simulink model "bike_model_v1_20190513_oldmodel"  (R2016b)
settings: Solver=ode23s  StartTime=0.0  StopTime=sim_time  FixedStep=Ts_IMU  MaxStep=Ts  RelTol=1e-3
values from neighbouring files (symbols this model uses):
  A = [0      0            1 ... (first row only)    [bike_init_v1_20190523_oldmodel_NOfeedback_RealModelComparison.m]    (also in bike_init_v1_20190524_oldmodel_positionfeedback_Nobalancing.m; bike_init_v1_20190527_oldmodel_NObalancing.m; bike_init_v1_20190527_oldmodel_positionfeedback_and_indicator.m; bike_init_v1_20190528_oldmodel_positionfeedback_and_indicator.m)
  B = [0; 1; (a_real*v*sin(lambda_real))/(h_real*b_real)]    [bike_init_v1_20190523_oldmodel_NOfeedback_RealModelComparison.m]    (also in bike_init_v1_20190524_oldmodel_positionfeedback_Nobalancing.m; bike_init_v1_20190527_oldmodel_NObalancing.m; bike_init_v1_20190527_oldmodel_positionfeedback_and_indicator.m; bike_init_v1_20190528_oldmodel_positionfeedback_and_indicator.m)
  b_model = 1.095*(1+(-0.1+(0.2*rand)))    [bike_init_v1_20190523_oldmodel_NOfeedback_RealModelComparison.m]    (also in bike_init_v1_20190524_oldmodel_positionfeedback_Nobalancing.m = 1.095; bike_init_v1_20190527_oldmodel_NObalancing.m = 1.095; bike_init_v1_20190527_oldmodel_positionfeedback_and_indicator.m = 1.095; bike_init_v1_20190528_oldmodel_positionfeedback_and_indicator.m = 1.095)
  b_real = 1.095    [bike_init_v1_20190523_oldmodel_NOfeedback_RealModelComparison.m]    (also in bike_init_v1_20190524_oldmodel_positionfeedback_Nobalancing.m; bike_init_v1_20190527_oldmodel_NObalancing.m; bike_init_v1_20190527_oldmodel_positionfeedback_and_indicator.m; bike_init_v1_20190528_oldmodel_positionfeedback_and_indicator.m)
  complementary = 0.985    [bike_init_v1_20190523_oldmodel_NOfeedback_RealModelComparison.m]    (also in bike_init_v1_20190524_oldmodel_positionfeedback_Nobalancing.m; bike_init_v1_20190527_oldmodel_NObalancing.m; bike_init_v1_20190527_oldmodel_positionfeedback_and_indicator.m; bike_init_v1_20190528_oldmodel_positionfeedback_and_indicator.m)
  cumulative_dist_along_path = [0;cumsum(dist_from_vertex_to_vertex,1)]    [bike_init_v1_20190523_oldmodel_NOfeedback_RealModelComparison.m]    (also in bike_init_v1_20190524_oldmodel_positionfeedback_Nobalancing.m; bike_init_v1_20190527_oldmodel_NObalancing.m; bike_init_v1_20190527_oldmodel_positionfeedback_and_indicator.m; bike_init_v1_20190528_oldmodel_positionfeedback_and_indicator.m)
  damp = 0.4    [bike_init_v1_20190523_oldmodel_NOfeedback_RealModelComparison.m]    (also in bike_init_v1_20190524_oldmodel_positionfeedback_Nobalancing.m; bike_init_v1_20190527_oldmodel_NObalancing.m; bike_init_v1_20190527_oldmodel_positionfeedback_and_indicator.m; bike_init_v1_20190528_oldmodel_positionfeedback_and_indicator.m)
  Dead_Band = [0.055,-0.055,0.005]    [bike_init_v1_20190523_oldmodel_NOfeedback_RealModelComparison.m]    (also in bike_init_v1_20190524_oldmodel_positionfeedback_Nobalancing.m; bike_init_v1_20190527_oldmodel_NObalancing.m; bike_init_v1_20190527_oldmodel_positionfeedback_and_indicator.m; bike_init_v1_20190528_oldmodel_positionfeedback_and_indicator.m)
  delay = 0.045    [bike_init_v1_20190523_oldmodel_NOfeedback_RealModelComparison.m]    (also in bike_init_v1_20190524_oldmodel_positionfeedback_Nobalancing.m; bike_init_v1_20190527_oldmodel_NObalancing.m; bike_init_v1_20190527_oldmodel_positionfeedback_and_indicator.m; bike_init_v1_20190528_oldmodel_positionfeedback_and_indicator.m)
  delta_control = 1    [bike_init_v1_20190523_oldmodel_NOfeedback_RealModelComparison.m]    (also in bike_init_v1_20190524_oldmodel_positionfeedback_Nobalancing.m; bike_init_v1_20190527_oldmodel_NObalancing.m; bike_init_v1_20190527_oldmodel_positionfeedback_and_indicator.m; bike_init_v1_20190528_oldmodel_positionfeedback_and_indicator.m)
  direct_control = 1    [bike_init_v1_20190523_oldmodel_NOfeedback_RealModelComparison.m]    (also in bike_init_v1_20190524_oldmodel_positionfeedback_Nobalancing.m; bike_init_v1_20190527_oldmodel_NObalancing.m; bike_init_v1_20190527_oldmodel_positionfeedback_and_indicator.m; bike_init_v1_20190528_oldmodel_positionfeedback_and_indicator.m)
  filter_model = 1    [bike_init_v1_20190523_oldmodel_NOfeedback_RealModelComparison.m]    (also in bike_init_v1_20190524_oldmodel_positionfeedback_Nobalancing.m; bike_init_v1_20190527_oldmodel_NObalancing.m; bike_init_v1_20190527_oldmodel_positionfeedback_and_indicator.m; bike_init_v1_20190528_oldmodel_positionfeedback_and_indicator.m)
  forward_motor_dynamics = 0    [bike_init_v1_20190523_oldmodel_NOfeedback_RealModelComparison.m]    (also in bike_init_v1_20190524_oldmodel_positionfeedback_Nobalancing.m; bike_init_v1_20190527_oldmodel_NObalancing.m; bike_init_v1_20190527_oldmodel_positionfeedback_and_indicator.m; bike_init_v1_20190528_oldmodel_positionfeedback_and_indicator.m)
  fr_oscil = 1    [bike_init_v1_20190523_oldmodel_NOfeedback_RealModelComparison.m]    (also in bike_init_v1_20190524_oldmodel_positionfeedback_Nobalancing.m; bike_init_v1_20190527_oldmodel_NObalancing.m; bike_init_v1_20190527_oldmodel_positionfeedback_and_indicator.m; bike_init_v1_20190528_oldmodel_positionfeedback_and_indicator.m)
  g = 9.81    [bike_init_v1_20190523_oldmodel_NOfeedback_RealModelComparison.m]    (also in bike_init_v1_20190524_oldmodel_positionfeedback_Nobalancing.m; bike_init_v1_20190527_oldmodel_NObalancing.m; bike_init_v1_20190527_oldmodel_positionfeedback_and_indicator.m; bike_init_v1_20190528_oldmodel_positionfeedback_and_indicator.m)
  gain = 0.3    [bike_init_v1_20190523_oldmodel_NOfeedback_RealModelComparison.m]    (also in bike_init_v1_20190524_oldmodel_positionfeedback_Nobalancing.m; bike_init_v1_20190527_oldmodel_NObalancing.m; bike_init_v1_20190527_oldmodel_positionfeedback_and_indicator.m; bike_init_v1_20190528_oldmodel_positionfeedback_and_indicator.m)
  IMU_height_model = 0.45*(1+(-0.1+(0.2*rand)))    [bike_init_v1_20190523_oldmodel_NOfeedback_RealModelComparison.m]    (also in bike_init_v1_20190524_oldmodel_positionfeedback_Nobalancing.m = 0.45; bike_init_v1_20190527_oldmodel_NObalancing.m = 0.45; bike_init_v1_20190527_oldmodel_positionfeedback_and_indicator.m = 0.45; bike_init_v1_20190528_oldmodel_positionfeedback_and_indicator.m = 0.45)
  IMU_height_real = 0.45    [bike_init_v1_20190523_oldmodel_NOfeedback_RealModelComparison.m]    (also in bike_init_v1_20190524_oldmodel_positionfeedback_Nobalancing.m; bike_init_v1_20190527_oldmodel_NObalancing.m; bike_init_v1_20190527_oldmodel_positionfeedback_and_indicator.m; bike_init_v1_20190528_oldmodel_positionfeedback_and_indicator.m)
  initial_states = [deg2rad(0) deg2rad(0) deg2rad(0)]    [bike_init_v1_20190523_oldmodel_NOfeedback_RealModelComparison.m]    (also in bike_init_v1_20190524_oldmodel_positionfeedback_Nobalancing.m; bike_init_v1_20190527_oldmodel_NObalancing.m; bike_init_v1_20190527_oldmodel_positionfeedback_and_indicator.m; bike_init_v1_20190528_oldmodel_positionfeedback_and_indicator.m = [deg2rad(1) deg2rad(0) deg2rad(0)])
  initial_x = path_x(1)+x_ini_diff    [bike_init_v1_20190523_oldmodel_NOfeedback_RealModelComparison.m]    (also in bike_init_v1_20190524_oldmodel_positionfeedback_Nobalancing.m; bike_init_v1_20190527_oldmodel_NObalancing.m; bike_init_v1_20190527_oldmodel_positionfeedback_and_indicator.m; bike_init_v1_20190528_oldmodel_positionfeedback_and_indicator.m)
  initial_y = radius+y_ini_diff    (= 20)    [bike_init_v1_20190523_oldmodel_NOfeedback_RealModelComparison.m]    (also in bike_init_v1_20190524_oldmodel_positionfeedback_Nobalancing.m; bike_init_v1_20190527_oldmodel_NObalancing.m; bike_init_v1_20190527_oldmodel_positionfeedback_and_indicator.m; bike_init_v1_20190528_oldmodel_positionfeedback_and_indicator.m)
  input_velocity = 2    [bike_init_v1_20190523_oldmodel_NOfeedback_RealModelComparison.m]    (also in bike_init_v1_20190524_oldmodel_positionfeedback_Nobalancing.m = 2.5; bike_init_v1_20190527_oldmodel_NObalancing.m = 2.5; bike_init_v1_20190527_oldmodel_positionfeedback_and_indicator.m = 3; bike_init_v1_20190528_oldmodel_positionfeedback_and_indicator.m = 7)
  K_full_dis = zeros(length(velocity_lqr),3)    [bike_init_v1_20190523_oldmodel_NOfeedback_RealModelComparison.m]    (also in bike_init_v1_20190524_oldmodel_positionfeedback_Nobalancing.m; bike_init_v1_20190527_oldmodel_NObalancing.m; bike_init_v1_20190527_oldmodel_positionfeedback_and_indicator.m; bike_init_v1_20190528_oldmodel_positionfeedback_and_indicator.m)
  lambda_model = deg2rad(70)*(1+(-0.1+(0.2*rand)))    [bike_init_v1_20190523_oldmodel_NOfeedback_RealModelComparison.m]    (also in bike_init_v1_20190524_oldmodel_positionfeedback_Nobalancing.m = deg2rad(70); bike_init_v1_20190527_oldmodel_NObalancing.m = deg2rad(70); bike_init_v1_20190527_oldmodel_positionfeedback_and_indicator.m = deg2rad(70); bike_init_v1_20190528_oldmodel_positionfeedback_and_indicator.m = deg2rad(70))
  lambda_real = deg2rad(70)    [bike_init_v1_20190523_oldmodel_NOfeedback_RealModelComparison.m]    (also in bike_init_v1_20190524_oldmodel_positionfeedback_Nobalancing.m; bike_init_v1_20190527_oldmodel_NObalancing.m; bike_init_v1_20190527_oldmodel_positionfeedback_and_indicator.m; bike_init_v1_20190528_oldmodel_positionfeedback_and_indicator.m)
  lat_control = 1    [bike_init_v1_20190523_oldmodel_NOfeedback_RealModelComparison.m]    (also in bike_init_v1_20190524_oldmodel_positionfeedback_Nobalancing.m; bike_init_v1_20190527_oldmodel_NObalancing.m; bike_init_v1_20190527_oldmodel_positionfeedback_and_indicator.m; bike_init_v1_20190528_oldmodel_positionfeedback_and_indicator.m)
  look_ahead = 0    [bike_init_v1_20190523_oldmodel_NOfeedback_RealModelComparison.m]    (also in bike_init_v1_20190524_oldmodel_positionfeedback_Nobalancing.m; bike_init_v1_20190527_oldmodel_NObalancing.m; bike_init_v1_20190527_oldmodel_positionfeedback_and_indicator.m; bike_init_v1_20190528_oldmodel_positionfeedback_and_indicator.m)
  max_handlebar = 40*(pi/180)    (= 0.698131700798)    [bike_init_v1_20190523_oldmodel_NOfeedback_RealModelComparison.m]    (also in bike_init_v1_20190524_oldmodel_positionfeedback_Nobalancing.m; bike_init_v1_20190527_oldmodel_NObalancing.m; bike_init_v1_20190527_oldmodel_positionfeedback_and_indicator.m; bike_init_v1_20190528_oldmodel_positionfeedback_and_indicator.m)
  max_roll = pi/2    (= 1.57079632679)    [bike_init_v1_20190523_oldmodel_NOfeedback_RealModelComparison.m]    (also in bike_init_v1_20190524_oldmodel_positionfeedback_Nobalancing.m; bike_init_v1_20190527_oldmodel_NObalancing.m; bike_init_v1_20190527_oldmodel_positionfeedback_and_indicator.m; bike_init_v1_20190528_oldmodel_positionfeedback_and_indicator.m)
  max_steering_motor_acc = inf    [bike_init_v1_20190523_oldmodel_NOfeedback_RealModelComparison.m]    (also in bike_init_v1_20190524_oldmodel_positionfeedback_Nobalancing.m; bike_init_v1_20190527_oldmodel_NObalancing.m; bike_init_v1_20190527_oldmodel_positionfeedback_and_indicator.m; bike_init_v1_20190528_oldmodel_positionfeedback_and_indicator.m)
  max_steering_motor_speed = 7.5    [bike_init_v1_20190523_oldmodel_NOfeedback_RealModelComparison.m]    (also in bike_init_v1_20190524_oldmodel_positionfeedback_Nobalancing.m; bike_init_v1_20190527_oldmodel_NObalancing.m; bike_init_v1_20190527_oldmodel_positionfeedback_and_indicator.m; bike_init_v1_20190528_oldmodel_positionfeedback_and_indicator.m)
  min_handlebar = -max_handlebar    (= -0.698131700798)    [bike_init_v1_20190523_oldmodel_NOfeedback_RealModelComparison.m]    (also in bike_init_v1_20190524_oldmodel_positionfeedback_Nobalancing.m; bike_init_v1_20190527_oldmodel_NObalancing.m; bike_init_v1_20190527_oldmodel_positionfeedback_and_indicator.m; bike_init_v1_20190528_oldmodel_positionfeedback_and_indicator.m)
  min_roll = - max_roll    (= -1.57079632679)    [bike_init_v1_20190523_oldmodel_NOfeedback_RealModelComparison.m]    (also in bike_init_v1_20190524_oldmodel_positionfeedback_Nobalancing.m; bike_init_v1_20190527_oldmodel_NObalancing.m; bike_init_v1_20190527_oldmodel_positionfeedback_and_indicator.m; bike_init_v1_20190528_oldmodel_positionfeedback_and_indicator.m)
  min_steering_motor_acc = -inf    [bike_init_v1_20190523_oldmodel_NOfeedback_RealModelComparison.m]    (also in bike_init_v1_20190524_oldmodel_positionfeedback_Nobalancing.m; bike_init_v1_20190527_oldmodel_NObalancing.m; bike_init_v1_20190527_oldmodel_positionfeedback_and_indicator.m; bike_init_v1_20190528_oldmodel_positionfeedback_and_indicator.m)
  min_steering_motor_speed = -7.5    [bike_init_v1_20190523_oldmodel_NOfeedback_RealModelComparison.m]    (also in bike_init_v1_20190524_oldmodel_positionfeedback_Nobalancing.m; bike_init_v1_20190527_oldmodel_NObalancing.m; bike_init_v1_20190527_oldmodel_positionfeedback_and_indicator.m; bike_init_v1_20190528_oldmodel_positionfeedback_and_indicator.m)
  noise = 1    [bike_init_v1_20190523_oldmodel_NOfeedback_RealModelComparison.m]    (also in bike_init_v1_20190524_oldmodel_positionfeedback_Nobalancing.m; bike_init_v1_20190527_oldmodel_NObalancing.m; bike_init_v1_20190527_oldmodel_positionfeedback_and_indicator.m; bike_init_v1_20190528_oldmodel_positionfeedback_and_indicator.m)
  noise_encoder = 1e-7    (= 1e-07)    [bike_init_v1_20190523_oldmodel_NOfeedback_RealModelComparison.m]    (also in bike_init_v1_20190524_oldmodel_positionfeedback_Nobalancing.m; bike_init_v1_20190527_oldmodel_NObalancing.m; bike_init_v1_20190527_oldmodel_positionfeedback_and_indicator.m; bike_init_v1_20190528_oldmodel_positionfeedback_and_indicator.m)
  noise_hall = 0    [bike_init_v1_20190523_oldmodel_NOfeedback_RealModelComparison.m]    (also in bike_init_v1_20190524_oldmodel_positionfeedback_Nobalancing.m = 0.01; bike_init_v1_20190527_oldmodel_NObalancing.m; bike_init_v1_20190527_oldmodel_positionfeedback_and_indicator.m = 0.01; bike_init_v1_20190528_oldmodel_positionfeedback_and_indicator.m = 0.01)
  oscillations_roll = 0    [bike_init_v1_20190523_oldmodel_NOfeedback_RealModelComparison.m]    (also in bike_init_v1_20190524_oldmodel_positionfeedback_Nobalancing.m; bike_init_v1_20190527_oldmodel_NObalancing.m; bike_init_v1_20190527_oldmodel_positionfeedback_and_indicator.m; bike_init_v1_20190528_oldmodel_positionfeedback_and_indicator.m)
  oscillations_steer = 0    [bike_init_v1_20190523_oldmodel_NOfeedback_RealModelComparison.m]    (also in bike_init_v1_20190524_oldmodel_positionfeedback_Nobalancing.m; bike_init_v1_20190527_oldmodel_NObalancing.m; bike_init_v1_20190527_oldmodel_positionfeedback_and_indicator.m; bike_init_v1_20190528_oldmodel_positionfeedback_and_indicator.m)
  parameters_model = [g h_model b_model a_model lambda_model c_model]    [bike_init_v1_20190523_oldmodel_NOfeedback_RealModelComparison.m]    (also in bike_init_v1_20190524_oldmodel_positionfeedback_Nobalancing.m; bike_init_v1_20190527_oldmodel_NObalancing.m; bike_init_v1_20190527_oldmodel_positionfeedback_and_indicator.m; bike_init_v1_20190528_oldmodel_positionfeedback_and_indicator.m)
  parameters_real = [g h_real b_real a_real lambda_real c_real]    [bike_init_v1_20190523_oldmodel_NOfeedback_RealModelComparison.m]    (also in bike_init_v1_20190524_oldmodel_positionfeedback_Nobalancing.m; bike_init_v1_20190527_oldmodel_NObalancing.m; bike_init_v1_20190527_oldmodel_positionfeedback_and_indicator.m; bike_init_v1_20190528_oldmodel_positionfeedback_and_indicator.m)
  path_tracking = 1    [bike_init_v1_20190523_oldmodel_NOfeedback_RealModelComparison.m]    (also in bike_init_v1_20190524_oldmodel_positionfeedback_Nobalancing.m; bike_init_v1_20190527_oldmodel_NObalancing.m; bike_init_v1_20190527_oldmodel_positionfeedback_and_indicator.m; bike_init_v1_20190528_oldmodel_positionfeedback_and_indicator.m = 0)
  path_x = [path_x1 path_x2 path_x3]    [bike_init_v1_20190523_oldmodel_NOfeedback_RealModelComparison.m]    (also in bike_init_v1_20190524_oldmodel_positionfeedback_Nobalancing.m; bike_init_v1_20190527_oldmodel_NObalancing.m; bike_init_v1_20190527_oldmodel_positionfeedback_and_indicator.m; bike_init_v1_20190528_oldmodel_positionfeedback_and_indicator.m)
  path_y = [path_y1 path_y2 path_y3]    [bike_init_v1_20190523_oldmodel_NOfeedback_RealModelComparison.m]    (also in bike_init_v1_20190524_oldmodel_positionfeedback_Nobalancing.m; bike_init_v1_20190527_oldmodel_NObalancing.m; bike_init_v1_20190527_oldmodel_positionfeedback_and_indicator.m; bike_init_v1_20190528_oldmodel_positionfeedback_and_indicator.m)
  plant_model = 1    [bike_init_v1_20190523_oldmodel_NOfeedback_RealModelComparison.m]    (also in bike_init_v1_20190524_oldmodel_positionfeedback_Nobalancing.m; bike_init_v1_20190527_oldmodel_NObalancing.m; bike_init_v1_20190527_oldmodel_positionfeedback_and_indicator.m; bike_init_v1_20190528_oldmodel_positionfeedback_and_indicator.m)
  roll_rate_coef = 0.9    [bike_init_v1_20190523_oldmodel_NOfeedback_RealModelComparison.m]    (also in bike_init_v1_20190524_oldmodel_positionfeedback_Nobalancing.m; bike_init_v1_20190527_oldmodel_NObalancing.m; bike_init_v1_20190527_oldmodel_positionfeedback_and_indicator.m; bike_init_v1_20190528_oldmodel_positionfeedback_and_indicator.m)
  sensordist = dout*pi/nrsensor    (= 0.439822971503)    [bike_init_v1_20190524_oldmodel_positionfeedback_Nobalancing.m]    (also in bike_init_v1_20190527_oldmodel_NObalancing.m; bike_init_v1_20190527_oldmodel_positionfeedback_and_indicator.m; bike_init_v1_20190528_oldmodel_positionfeedback_and_indicator.m; bike_init_v1_20190531_oldmodel_positionfeedback_and_indicator.m)
  steering_motor_limitations = 1    [bike_init_v1_20190523_oldmodel_NOfeedback_RealModelComparison.m]    (also in bike_init_v1_20190524_oldmodel_positionfeedback_Nobalancing.m; bike_init_v1_20190527_oldmodel_NObalancing.m; bike_init_v1_20190527_oldmodel_positionfeedback_and_indicator.m; bike_init_v1_20190528_oldmodel_positionfeedback_and_indicator.m)
  sys_con = ss(A,B,C,D)    [bike_init_v1_20190523_oldmodel_NOfeedback_RealModelComparison.m]    (also in bike_init_v1_20190524_oldmodel_positionfeedback_Nobalancing.m; bike_init_v1_20190527_oldmodel_NObalancing.m; bike_init_v1_20190527_oldmodel_positionfeedback_and_indicator.m; bike_init_v1_20190528_oldmodel_positionfeedback_and_indicator.m)
  sys_dis = c2d(sys_con,Ts)    [bike_init_v1_20190523_oldmodel_NOfeedback_RealModelComparison.m]    (also in bike_init_v1_20190524_oldmodel_positionfeedback_Nobalancing.m; bike_init_v1_20190527_oldmodel_NObalancing.m; bike_init_v1_20190527_oldmodel_positionfeedback_and_indicator.m; bike_init_v1_20190528_oldmodel_positionfeedback_and_indicator.m)
  ToleranceVelocityEst = 0.5    [bike_init_v1_20190524_oldmodel_positionfeedback_Nobalancing.m]    (also in bike_init_v1_20190527_oldmodel_NObalancing.m; bike_init_v1_20190527_oldmodel_positionfeedback_and_indicator.m; bike_init_v1_20190528_oldmodel_positionfeedback_and_indicator.m; bike_init_v1_20190531_oldmodel_positionfeedback_and_indicator.m)
  Ts = 0.04    [bike_init_v1_20190523_oldmodel_NOfeedback_RealModelComparison.m]    (also in bike_init_v1_20190524_oldmodel_positionfeedback_Nobalancing.m; bike_init_v1_20190527_oldmodel_NObalancing.m; bike_init_v1_20190527_oldmodel_positionfeedback_and_indicator.m; bike_init_v1_20190528_oldmodel_positionfeedback_and_indicator.m)
  Ts_IMU = 0.04    [bike_init_v1_20190523_oldmodel_NOfeedback_RealModelComparison.m]    (also in bike_init_v1_20190524_oldmodel_positionfeedback_Nobalancing.m; bike_init_v1_20190527_oldmodel_NObalancing.m; bike_init_v1_20190527_oldmodel_positionfeedback_and_indicator.m; bike_init_v1_20190528_oldmodel_positionfeedback_and_indicator.m)
  velocity_lqr = [velocity_lqr-0.1 velocity_lqr velocity_lqr+0.1]    [bike_init_v1_20190523_oldmodel_NOfeedback_RealModelComparison.m]    (also in bike_init_v1_20190524_oldmodel_positionfeedback_Nobalancing.m; bike_init_v1_20190527_oldmodel_NObalancing.m; bike_init_v1_20190527_oldmodel_positionfeedback_and_indicator.m; bike_init_v1_20190528_oldmodel_positionfeedback_and_indicator.m)
  velocity_wave_amp = 0.5    [bike_init_v1_20190523_oldmodel_NOfeedback_RealModelComparison.m]    (also in bike_init_v1_20190524_oldmodel_positionfeedback_Nobalancing.m; bike_init_v1_20190527_oldmodel_NObalancing.m; bike_init_v1_20190527_oldmodel_positionfeedback_and_indicator.m; bike_init_v1_20190528_oldmodel_positionfeedback_and_indicator.m)
  velocity_wave_freq = 0.3*2*pi    (= 1.88495559215)    [bike_init_v1_20190523_oldmodel_NOfeedback_RealModelComparison.m]    (also in bike_init_v1_20190524_oldmodel_positionfeedback_Nobalancing.m; bike_init_v1_20190527_oldmodel_NObalancing.m; bike_init_v1_20190527_oldmodel_positionfeedback_and_indicator.m; bike_init_v1_20190528_oldmodel_positionfeedback_and_indicator.m)
undefined symbols (not defined in the file or in its folder): curvature
libraries: simulink x13, dspsigops x2, simulink_extras x1
(part 3 of 3)

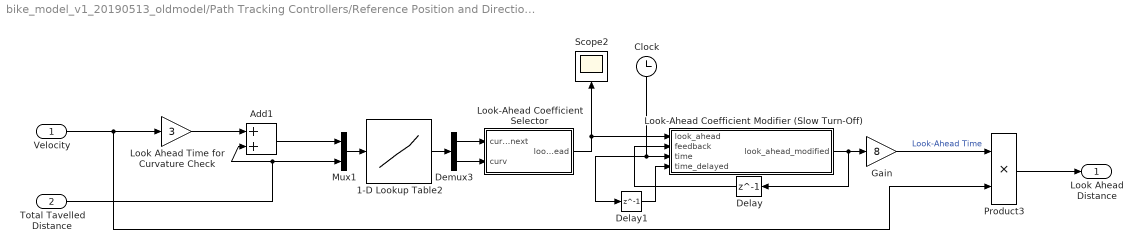
== system bike_model_v1_20190513_oldmodel/Path Tracking Controllers/Reference Position and Direction in Global CS with variable Look Ahead/Variable Look Ahead ==
  Velocity : Inport
  Total Tavelled Distance : Inport  Port=2
  1-D Lookup Table2 : Lookup_n-D  NumberOfTableDimensions=1  BreakpointsForDimension1=cumulative_dist_along_path  Table=curvature  ExtrapMethod=Clip  DiagnosticForOutOfRangeInput=Error  InternalRulePriority=Speed  RndMeth=Simplest  InputSameDT=on
  Add1 : Sum
  Clock : Clock
  Delay : Delay  DelayLength=1
  Delay1 : Delay  DelayLength=1
  Demux3 : Demux  Outputs=2
  Gain : Gain  Gain=8
  Look Ahead Time for Curvature Check : Gain  Gain=3
  Look-Ahead Coefficient Selector : MATLAB Function  TreatAsAtomicUnit=on
  "Look-Ahead Coefficient Modifier (Slow Turn-Off) " : MATLAB Function  TreatAsAtomicUnit=on
  Mux1 : Mux  Inputs=2
  Product3 : Product
  Scope2 : Scope
  Look Ahead Distance : Outport
  wires:
  Look Ahead Time for Curvature Check/1 -> Add1/1
  Delay/1 -> "Look-Ahead Coefficient Modifier (Slow Turn-Off) "/2(feedback)
  "Look-Ahead Coefficient Modifier (Slow Turn-Off) "/1(look_ahead_modified) -> Delay/1, Gain/1
  Demux3/1 -> Look-Ahead Coefficient Selector/1(curv_next)
  Look-Ahead Coefficient Selector/1(look_ahead) -> "Look-Ahead Coefficient Modifier (Slow Turn-Off) "/1(look_ahead), Scope2/1
  Clock/1 -> "Look-Ahead Coefficient Modifier (Slow Turn-Off) "/3(time), Delay1/1
  Delay1/1 -> "Look-Ahead Coefficient Modifier (Slow Turn-Off) "/4(time_delayed)
  1-D Lookup Table2/1 -> Demux3/1
  Total Tavelled Distance/1 -> Add1/2, Mux1/2
  Demux3/2 -> Look-Ahead Coefficient Selector/2(curv)
  Gain/1 -> Product3/1  "Look-Ahead Time"
  Add1/1 -> Mux1/1
  Mux1/1 -> 1-D Lookup Table2/1
  Velocity/1 -> Product3/2, Look Ahead Time for Curvature Check/1
  Product3/1 -> Look Ahead Distance/1

== system bike_model_v1_20190513_oldmodel/Complementary filter/Roll Angle Estimation of Accelerometer/Lateral Acceleration Compensator/Low Pass Filter ==
  Roll Rate : Inport
  Delay18 : Delay  DelayLength=1
  Gain4 : Gain  Gain=roll_rate_coef
  Gain6 : Gain  Gain=1-roll_rate_coef
  Scope7 : Scope  NumInputPorts=2
  Sum4 : Sum  Inputs=|++
  Filtered Roll Rate : Outport
  wires:
  Gain6/1 -> Sum4/1
  Gain4/1 -> Sum4/2
  Sum4/1 -> Filtered Roll Rate/1, Delay18/1, Scope7/2  "Filtered Roll Rate"
  Delay18/1 -> Gain4/1
  Roll Rate/1 -> Scope7/1, Gain6/1  "Measured Roll Rate"

== system bike_model_v1_20190513_oldmodel/Complementary filter/Roll Angle Estimation of Accelerometer/Lateral Acceleration Compensator/Numerical Derivative ==
  Roll Rate : Inport
  Delay18 : Delay  DelayLength=1
  Gain3 : Gain  Gain=1/Ts_IMU
  Sum3 : Sum  Inputs=|+-
  Roll Acceleration : Outport
  wires:
  Sum3/1 -> Gain3/1
  Delay18/1 -> Sum3/2
  Roll Rate/1 -> Sum3/1, Delay18/1
  Gain3/1 -> Roll Acceleration/1

== system bike_model_v1_20190513_oldmodel/Complementary filter/Roll Angle Estimation of Accelerometer/Lateral Acceleration Compensator/Subsystem ==
  In1 : Inport
  Constant : Constant  Value=A
  Constant1 : Constant  Value=B
  Delay1 : Delay  DelayLength=1  InitialCondition=[0 0 0]  SampleTime=Ts_IMU
  Multiply : Product  Multiplication=Matrix(*)
  Multiply1 : Product  Multiplication=Matrix(*)
  Sum2 : Sum  Inputs=|++
  Out1 : Outport
  wires:
  Sum2/1 -> Delay1/1
  Multiply1/1 -> Sum2/2
  In1/1 -> Multiply1/2  "u"
  Delay1/1 -> Multiply/2, Out1/1  "x"
  Multiply/1 -> Sum2/1
  Constant/1 -> Multiply/1
  Constant1/1 -> Multiply1/1

== matlab function bike_model_v1_20190513_oldmodel/Balance Controller/Reference States/Reference Roll Angle Calculator ==
  data: parameters_real input; velocity input; delta_ref input; phi_ref output
function phi_ref = fcn(parameters_real, velocity, delta_ref)
g = parameters_real(1);
b = parameters_real(3);
v = velocity;

phi_ref = -atan(v^2 / (g * b) * delta_ref); % tan(theta_ref));

== matlab function bike_model_v1_20190513_oldmodel/Physical Bike/Linear Bicycle Model ==
  data: states input; input input; xdot output; velocity input; disturbance input; parameters_real input
function xdot = fcn(states,input,velocity,disturbance,parameters_real)

delta_d=input;
v=velocity;
d1=disturbance(1);
d2=disturbance(2);
d3=disturbance(3);

g=parameters_real(1);
h=parameters_real(2);
b=parameters_real(3);
a=parameters_real(4);
lambda=parameters_real(5);
c=parameters_real(6);

phi=states(1);
delta=states(2);
phi_d=states(3);

xdot1=phi_d+d1;
xdot2=delta_d+d2;
xdot3=(g/h)*phi+((a*v)/(b*h))*sin(lambda)*delta_d+((h*v^2-g*a*c)/(b*h^2))*sin(lambda)*delta+d3;

xdot=[xdot1 xdot2 xdot3];

== matlab function bike_model_v1_20190513_oldmodel/Global Angles and Coordinates Calculator/Measured Bike Angles to Global Angles/MATLAB Function ==
  data: v input; parameters_model input; delta input; psi_d output; beta output
function [psi_d, beta]  = fcn(v, parameters_model, delta)

b = parameters_model(3);
a = parameters_model(4);

beta = atan((a / (b)) * tan(delta));
psi_d = (v / a) * sin(beta);

== matlab function bike_model_v1_20190513_oldmodel/Path Tracking Controllers/Reference Position and Direction in Global CS with variable Look Ahead/Variable Look Ahead/Look-Ahead Coefficient Modifier (Slow Turn-Off)  ==
  data: look_ahead input; look_ahead_modified output; feedback input; time input; time_delayed input
function look_ahead_modified = fcn(look_ahead, feedback, time, time_delayed)

step=time-time_delayed;

kill_time=3;

delta=(feedback*step)/kill_time;

if look_ahead-feedback<-0.0001
    look_ahead_modified=feedback-delta;
else
    look_ahead_modified = look_ahead;
end
    

end

== matlab function bike_model_v1_20190513_oldmodel/Global Angles and Coordinates Calculator/Measured Global Angles to Global Coordinates/MATLAB Function1 ==
  data: v input; psi input; Xdot output; beta input; Ydot output
function [Xdot, Ydot]  = fcn(v, psi, beta)

Xdot = v * cos(psi + beta);
Ydot = v * sin(psi + beta);

== matlab function bike_model_v1_20190513_oldmodel/Path Tracking Controllers/Reference Position and Direction in Global CS with variable Look Ahead/Variable Look Ahead/Look-Ahead Coefficient Selector ==
  data: curv_next input; look_ahead output; curv input
function look_ahead = fcn(curv_next, curv)


if curv>-0.01 && curv<0.01
    curv=0;
end

if curv_next>-0.01 && curv_next<0.01
    curv_next=0;
end



if curv>=0
    if curv-curv_next>0
        look_ahead=0;
    else
        look_ahead=curv_next-curv;
    end
else
    if curv-curv_next<0
        look_ahead=0;
    else
        look_ahead=curv-curv_next;
    end
end



end

== matlab function bike_model_v1_20190513_oldmodel/Complementary filter/Roll Angle Estimation of Accelerometer/Lateral Acceleration Compensator/Linear Bicycle Model ==
  data: states input; input input; xdot output; velocity input; parameters_model input
function xdot = fcn(states,input,velocity,parameters_model)

delta_d=input;
v=velocity;

g=parameters_model(1);
h=parameters_model(2);
b=parameters_model(3);
a=parameters_model(4);
lambda=parameters_model(5);
c=parameters_model(6);

phi=states(1);
delta=states(2);
phi_d=states(3);

xdot1=phi_d;
xdot2=delta_d;
xdot3=(g/h)*phi+((a*v)/(b*h))*sin(lambda)*delta_d+((h*v^2-g*a*c)/(b*h^2))*sin(lambda)*delta;

xdot=[xdot1 xdot2 xdot3];

== matlab function bike_model_v1_20190513_oldmodel/Global Angles and Coordinates Calculator/True Bike Angles to Global Angles2/MATLAB Function ==
  data: v input; parameters_real input; delta input; psi_d output; beta output
function [psi_d, beta]  = fcn(v, parameters_real, delta)

b = parameters_real(3);
a = parameters_real(4);

beta = atan((a / (b)) * tan(delta));
psi_d = (v / a) * sin(beta);

== matlab function bike_model_v1_20190513_oldmodel/Global Angles and Coordinates Calculator/True Global Angles to Global Coordinates/MATLAB Function1 ==
  data: v input; psi input; Xdot output; beta input; Ydot output
function [Xdot, Ydot]  = fcn(v, psi, beta)

Xdot = v * cos(psi + beta);
Ydot = v * sin(psi + beta);

== matlab function bike_model_v1_20190513_oldmodel/Physical Bike/Nonlinear Bicycle Model ==
  data: states input; input input; xdot output; velocity input; disturbance input; parameters_real input
function xdot = fcn(states,input,velocity,disturbance,parameters_real)

delta_d=input;
v=velocity;
d1=disturbance(1);
d2=disturbance(2);
d3=disturbance(3);

g=parameters_real(1);
h=parameters_real(2);
b=parameters_real(3);
a=parameters_real(4);
lambda=parameters_real(5);
c=parameters_real(6);

phi=states(1);
delta=states(2);
phi_d=states(3);

xdot1=phi_d+d1;
xdot2=delta_d+d2;
xdot3=(g/h)*tan(phi)+((a*v)/(b*h))*sin(lambda)*tan(delta_d)+((h*v^2-g*a*c)/(b*h^2))*sin(lambda)*tan(delta)+d3;

xdot=[xdot1 xdot2 xdot3];

== matlab function bike_model_v1_20190513_oldmodel/Physical Bike/Linear Bicycle Model with neglected fork angle (lambda=90deg, c=0) "THE SIMPLEST MODEL" ==
  data: states input; input input; xdot output; velocity input; disturbance input; parameters_real input
function xdot = fcn(states,input,velocity,disturbance,parameters_real)

delta_d=input;
v=velocity;
d1=disturbance(1);
d2=disturbance(2);
d3=disturbance(3);

g=parameters_real(1);
h=parameters_real(2);
b=parameters_real(3);
a=parameters_real(4);

phi=states(1);
delta=states(2);
phi_d=states(3);

xdot1=phi_d+d1;
xdot2=delta_d+d2;
xdot3=(g/h)*phi+((a*v)/(b*h))*delta_d+((v^2)/(b*h))*delta+d3;

xdot=[xdot1 xdot2 xdot3];

== matlab function bike_model_v1_20190513_oldmodel/Complementary filter/Roll Angle Estimation of Accelerometer/Lateral Acceleration Compensator/Linear Bicycle Model1 ==
  data: states input; input input; xdot output; velocity input; parameters_model input
function xdot = fcn(states,input,velocity,parameters_model)

delta_d=input;
v=velocity;

g=parameters_model(1);
h=parameters_model(2);
b=parameters_model(3);
a=parameters_model(4);
lambda=parameters_model(5);
c=parameters_model(6);

phi=states(1);
delta=states(2);
phi_d=states(3);

xdot1=phi_d;
xdot2=delta_d;
xdot3=(g/h)*phi+((a*v)/(b*h))*sin(lambda)*delta_d+((h*v^2-g*a*c)/(b*h^2))*sin(lambda)*delta;

xdot=[xdot1; xdot2; xdot3];

== matlab function bike_model_v1_20190513_oldmodel/Complementary filter/Roll Angle Estimation of Accelerometer/Lateral Acceleration Compensator/discrete ==
  data: states input; input input; x_next output; A input; B input
function x_next = fcn(states,input,A,B)





x_next=A*states+B*input;

== matlab function bike_model_v1_20190513_oldmodel/Hall Sensor Ver2/MATLAB Function ==
  settings: updateMethod=DISCRETE
  data: Dist input; Vout output; hallsensor_dist input; count input; Pulse output; newcount_output output; T input
function [Vout,Pulse, newcount_output] = fcn(Dist, hallsensor_dist, count, T)
persistent Vmemory T0 correctrate PulseFlag DropRate realcount
coder.extrinsic('exist')

if(isempty(Vmemory))
    Vmemory = 0;
%     correctrate = 1-0.001;
    DropRate = 1-0.01;
    T0 = T;
    realcount = 0;
end

Newcount = floor(Dist/hallsensor_dist);
if Newcount >= realcount+1
    PulseFlag = 1;
    realcount = Newcount;
    if (rand/DropRate)>1
        PulseFlag = 0;
    end

    if PulseFlag == 1
        dT = T - T0;
        T0 = T;
        Vmemory = hallsensor_dist/dT;
        Pulse = 1;
        PulseFlag = 0;
        newcount_output = count + 1;
    else
        Pulse = 0;
        newcount_output = count;
    end
    Vout = Vmemory; 
else
    if  T - T0> 0.65
        Vmemory = 0;
    end
    Vout = Vmemory;
    Pulse = 0;
    newcount_output = count;
    PulseFlag = 0;
end

% IF YOU WANT TO ADD RANDOM VELOCITY READING DROP, YOU CAN UNCOMMENT THIS
% % if(rand/correctrate)>1
% %     Vout = Vmemory * rand;
% %     Vmemory = Vout;
% % end

end

== matlab function bike_model_v1_20190513_oldmodel/Hall Sensor Ver2/MATLAB Function1 ==
  data: Dist input; Pulse output; SensorDist input; PulseAccept input
function Pulse = PulseGen(Dist,SensorDist, PulseAccept)
persistent Count 
if(isempty(Count))
    Count = 0;
end

Newcount = floor(Dist/hallsensor_dist);
if Newcount >= count+1
    dT = T - T0;
    T0 = T;
    vold = Vmemory;
    Vmemory = hallsensor_dist/dT;
    Vout = Vmemory;
    Pulse = 1;
    newcount = Newcount;
    
%     if(rand/correctrate)>1
%         T0 = T0 - dT;
%         Vmemory = vold;
%         Pulse = 0;
%         newcount = Newcount-1;
%     end
    
else
    Vout = Vmemory;
    Pulse = 0;
    newcount = Newcount;
end

y = u;

== matlab function bike_model_v1_20190513_oldmodel/Hall Sensor Ver2/MATLAB Function2 ==
  settings: updateMethod=DISCRETE
  data: Dist input; Vout output; hallsensor_dist input; count input; Pulse output; newcount output; T input
function [Vout,Pulse, newcount] = fcnVer2(Dist, hallsensor_dist, count, T)
persistent Vmemory T0 correctrate
coder.extrinsic('exist')

if(isempty(Vmemory))
    Vmemory = 0;
    correctrate = 1-0.001;
end
if(isempty(T0))
    T0 = T;
%     newcount = 0;
%     Pulse = 0;
end
Newcount = floor(Dist/hallsensor_dist);
if Newcount >= count+1
    dT = T - T0;
    T0 = T;
    vold = Vmemory;
    Vmemory = hallsensor_dist/dT;
    Vout = Vmemory;
    Pulse = 1;
    newcount = Newcount;
    
%     if(rand/correctrate)>1
%         T0 = T0 - dT;
%         Vmemory = vold;
%         Pulse = 0;
%         newcount = Newcount-1;
%     end
    
else
    Vout = Vmemory;
    Pulse = 0;
    newcount = Newcount;
end

if(rand/correctrate)>1
    Vout = Vmemory * rand;
    Vmemory = Vout;
end

end

== matlab function bike_model_v1_20190513_oldmodel/HallSensor Filter/Complementary Filter Hall Sensor ==
  data: HalVel input; EstimatedVelocity output; PulseCount input; Accx input; T input; Toler input
function EstimatedVelocity = complementaryfilterHallSensor(HalVel,PulseCount,Accx,T,Toler)
% The function is based on Umur's thesis 3.1, where acc_x corresponds to
% \dot{v}, however, I haven't calculated and proved this, So Be Cautious
% that, this only hold for flat ground, and the correctness is
% suspective...
persistent OldCount Vel OldVel
coder.extrinsic('warning')
if(isempty(OldCount))
    OldCount = 0;
    Vel = 0;
    OldVel = 0;
end
if PulseCount > OldCount % The HalVel value has been updated
        OldCount = PulseCount;
    if ((HalVel > Vel + Toler) || (HalVel < Vel - Toler)) && (OldCount > 2) % If not braked, the hall sensor starts making error
        disp('The hall sensor error has been detected')
        Vel = Vel + Accx*T;
    else
        Vel = HalVel;
    end

elseif (PulseCount == OldCount) ||(HalVel == OldVel) % When the velocity of hall sensor is not updated, while redundent
    Vel = Vel + Accx*T;
else
    warning('Strange Case happens in Hallsensor velocity filter, check it!')
end
EstimatedVelocity = Vel;
end
